simulink model "Subsystem"  (R2024a)
settings: Solver=VariableStepAuto  StartTime=0.0  StopTime=10.0  RelTol=1e-3
libraries: simulink x4
settings Model: Creator=50803  LastModifiedBy=50803

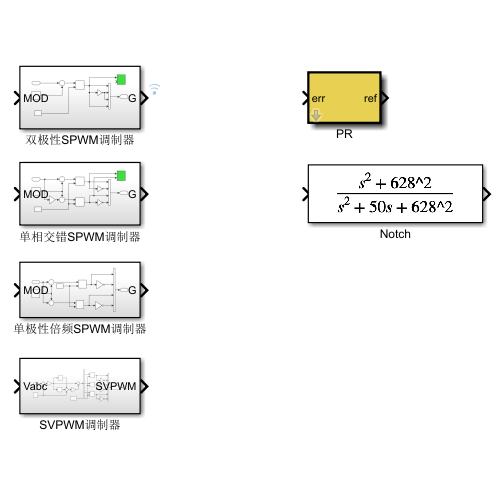
[thumbnail: Simulink's stored preview of the top-level diagram]
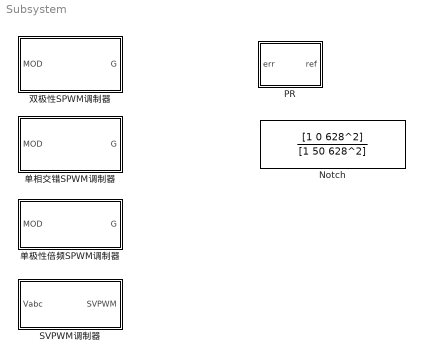
== system Subsystem ==
  Notch : TransferFcn  Numerator=[1 0 628^2]  Denominator=[1 50 628^2]
  PR : Subsystem  TreatAsAtomicUnit=on  mask{Kp=2, Kr=100, Wc=5, Upper=1200, Lower=-1200}
  SVPWM调制器 : Subsystem
  单极性倍频SPWM调制器 : Subsystem
  单相交错SPWM调制器 : Subsystem
  双极性SPWM调制器 : Subsystem

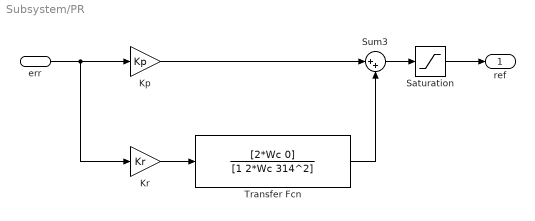
== system Subsystem/PR ==
  err : Inport
  Kp : Gain  Gain=Kp
  Kr : Gain  Gain=Kr
  Saturation : Saturate  UpperLimit=Upper  LowerLimit=Lower
  Sum3 : Sum  Inputs=|++
  Transfer Fcn : TransferFcn  Numerator=[2*Wc 0]  Denominator=[1 2*Wc 314^2]
  ref : Outport
  wires:
  Kp/1 -> Sum3/1
  Sum3/1 -> Saturation/1
  err/1 -> Kr/1, Kp/1
  Kr/1 -> Transfer Fcn/1
  Transfer Fcn/1 -> Sum3/2
  Saturation/1 -> ref/1

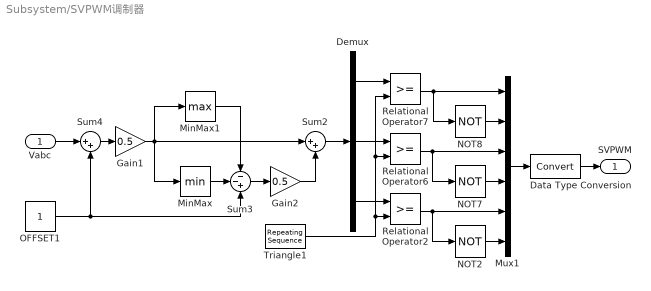
== system Subsystem/SVPWM调制器 ==
  Vabc : Inport
  Data Type Conversion : DataTypeConversion  SaturateOnIntegerOverflow=off  RndMeth=Floor
  Demux : Demux  Outputs=3
  Gain1 : Gain  Gain=0.5
  Gain2 : Gain  Gain=0.5
  MinMax : MinMax
  MinMax1 : MinMax  Function=max
  Mux1 : Mux  Inputs=6
  NOT2 : Logic  Operator=NOT  IconShape=distinctive  AllPortsSameDT=off  OutDataTypeStr=boolean
  NOT7 : Logic  Operator=NOT  IconShape=distinctive  AllPortsSameDT=off  OutDataTypeStr=boolean
  NOT8 : Logic  Operator=NOT  IconShape=distinctive  AllPortsSameDT=off  OutDataTypeStr=boolean
  OFFSET1 : Constant
  Relational Operator2 : RelationalOperator  OutDataTypeStr=boolean  InputSameDT=off
  Relational Operator6 : RelationalOperator  OutDataTypeStr=boolean  InputSameDT=off
  Relational Operator7 : RelationalOperator  OutDataTypeStr=boolean  InputSameDT=off
  Sum2 : Sum  Inputs=|++
  Sum3 : Sum  Inputs=--+
  Sum4 : Sum  Inputs=|++
  Triangle1 : simulink/Sources/Repeating Sequence  rep_seq_t=[0 1/20000/2 1/20000]  rep_seq_y=[0 1 0]
  SVPWM : Outport
  wires:
  Gain2/1 -> Sum2/2
  Relational Operator6/1 -> Mux1/3, NOT7/1
  NOT7/1 -> Mux1/4
  Relational Operator7/1 -> Mux1/1, NOT8/1
  Triangle1/1 -> Relational Operator2/2, Relational Operator7/2, Relational Operator6/2
  NOT8/1 -> Mux1/2
  Gain1/1 -> MinMax/1, MinMax1/1, Sum2/1
  Relational Operator2/1 -> Mux1/5, NOT2/1
  NOT2/1 -> Mux1/6
  Vabc/1 -> Sum4/1
  OFFSET1/1 -> Sum4/2, Sum3/3
  Sum4/1 -> Gain1/1
  Sum3/1 -> Gain2/1
  MinMax/1 -> Sum3/2
  MinMax1/1 -> Sum3/1
  Demux/1 -> Relational Operator7/1
  Demux/2 -> Relational Operator6/1
  Demux/3 -> Relational Operator2/1
  Sum2/1 -> Demux/1
  Mux1/1 -> Data Type Conversion/1
  Data Type Conversion/1 -> SVPWM/1

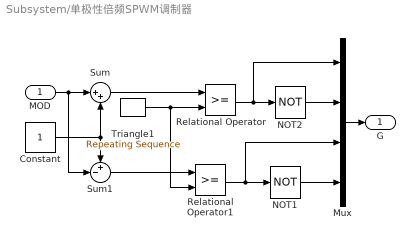
== system Subsystem/单极性倍频SPWM调制器 ==
  MOD : Inport
  Constant : Constant
  Mux : Mux
  NOT1 : Logic  Operator=NOT  IconShape=distinctive  AllPortsSameDT=off  OutDataTypeStr=boolean
  NOT2 : Logic  Operator=NOT  IconShape=distinctive  AllPortsSameDT=off  OutDataTypeStr=boolean
  Relational Operator : RelationalOperator  OutDataTypeStr=boolean  RndMeth=Simplest  InputSameDT=off
  Relational Operator1 : RelationalOperator  OutDataTypeStr=boolean  RndMeth=Simplest  InputSameDT=off
  Sum : Sum  Inputs=|++
  Sum1 : Sum  Inputs=+-|
  Triangle1 : simulink/Sources/Repeating Sequence  rep_seq_t=[0 1/20000/2 1/20000]  rep_seq_y=[0 2 0]
  G : Outport
  wires:
  MOD/1 -> Sum1/2, Sum/1
  Mux/1 -> G/1
  Constant/1 -> Sum/2, Sum1/1
  Sum/1 -> Relational Operator/1
  Triangle1/1 -> Relational Operator1/2, Relational Operator/2
  Relational Operator/1 -> NOT2/1, Mux/1
  Sum1/1 -> Relational Operator1/1
  Relational Operator1/1 -> Mux/3, NOT1/1
  NOT1/1 -> Mux/4
  NOT2/1 -> Mux/2

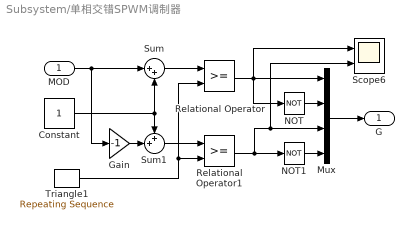
== system Subsystem/单相交错SPWM调制器 ==
  MOD : Inport
  Constant : Constant
  Gain : Gain  Gain=-1
  Mux : Mux
  NOT : Logic  Operator=NOT  IconShape=distinctive  AllPortsSameDT=off  OutDataTypeStr=boolean
  NOT1 : Logic  Operator=NOT  IconShape=distinctive  AllPortsSameDT=off  OutDataTypeStr=boolean
  Relational Operator : RelationalOperator  OutDataTypeStr=boolean  InputSameDT=off
  Relational Operator1 : RelationalOperator  OutDataTypeStr=boolean  InputSameDT=off
  Scope6 : Scope  NumInputPorts=2
  Sum : Sum  Inputs=|++
  Sum1 : Sum  Inputs=++|
  Triangle1 : simulink/Sources/Repeating Sequence  rep_seq_t=[0 1/30000/2 1/30000]  rep_seq_y=[0 2 0]
  G : Outport
  wires:
  Triangle1/1 -> Relational Operator1/2, Relational Operator/2
  Mux/1 -> G/1
  NOT/1 -> Mux/2
  Relational Operator/1 -> Scope6/1, Mux/1, NOT/1
  MOD/1 -> Sum/1, Gain/1
  Sum/1 -> Relational Operator/1
  Sum1/1 -> Relational Operator1/1
  Relational Operator1/1 -> Scope6/2, Mux/3, NOT1/1
  Constant/1 -> Sum1/1, Sum/2
  Gain/1 -> Sum1/2
  NOT1/1 -> Mux/4

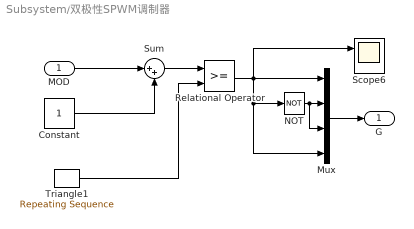
== system Subsystem/双极性SPWM调制器 ==
  MOD : Inport
  Constant : Constant
  Mux : Mux
  NOT : Logic  Operator=NOT  IconShape=distinctive  AllPortsSameDT=off  OutDataTypeStr=boolean
  Relational Operator : RelationalOperator  OutDataTypeStr=boolean  InputSameDT=off
  Scope6 : Scope  NumInputPorts=2
  Sum : Sum  Inputs=|++
  Triangle1 : simulink/Sources/Repeating Sequence  rep_seq_t=[0 1/30000/2 1/30000]  rep_seq_y=[0 2 0]
  G : Outport
  wires:
  Constant/1 -> Sum/2
  Sum/1 -> Relational Operator/1
  MOD/1 -> Sum/1
  Relational Operator/1 -> NOT/1, Mux/4, Mux/1, Scope6/1
  NOT/1 -> Mux/2, Mux/3
  Mux/1 -> G/1
  Triangle1/1 -> Relational Operator/2
